simulink model "ProcessAttitude"  (R2018b)
settings: configuration reference "RPi_ControlRate" (kept outside this file)
values from neighbouring files (symbols this model uses):
  rangeTable = [2500 5000]    [loadSensorData.m]
settings Model: Creator=barthal  LastModifiedBy=barthal
settings ConfigSetRef: SourceLocation=Base Workspace

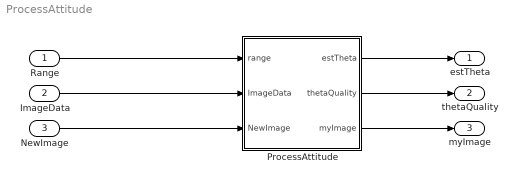
== system ProcessAttitude ==
  Range : Inport
  ImageData : Inport  Port=2  OutDataTypeStr=uint8
  NewImage : Inport  Port=3  OutDataTypeStr=uint8
  ProcessAttitude : Subsystem
  estTheta : Outport
  thetaQuality : Outport  Port=2
  myImage : Outport  Port=3  OutDataTypeStr=uint8
  wires:
  ImageData/1 -> ProcessAttitude/2(ImageData)
  Range/1 -> ProcessAttitude/1(range)
  ProcessAttitude/1(estTheta) -> estTheta/1
  ProcessAttitude/2(thetaQuality) -> thetaQuality/1
  ProcessAttitude/3(myImage) -> myImage/1
  NewImage/1 -> ProcessAttitude/3(NewImage)

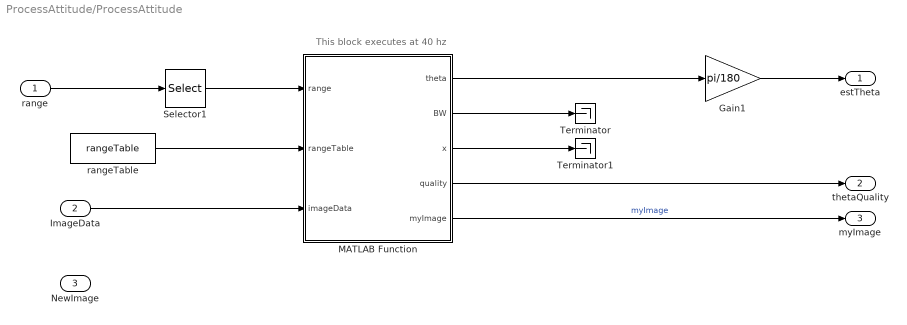
== system ProcessAttitude/ProcessAttitude ==
  note: This block executes at 40 hz
  range : Inport  PortDimensions=4
  ImageData : Inport  Port=2  OutDataTypeStr=uint8  PortDimensions=[307200]
  NewImage : Inport  Port=3
  Gain1 : Gain  Gain=pi/180
  MATLAB Function : MATLAB Function  TreatAsAtomicUnit=on
  Selector1 : Selector  InputPortWidth=4  IndexOptions=Index vector (dialog)  Indices=1  OutputSizes=1
  Terminator : Terminator
  Terminator1 : Terminator
  rangeTable : Constant  Value=rangeTable
  estTheta : Outport
  thetaQuality : Outport  Port=2
  myImage : Outport  Port=3  OutDataTypeStr=uint8
  wires:
  MATLAB Function/3(x) -> Terminator1/1
  MATLAB Function/2(BW) -> Terminator/1
  MATLAB Function/5(myImage) -> myImage/1  "myImage"
  MATLAB Function/4(quality) -> thetaQuality/1
  MATLAB Function/1(theta) -> Gain1/1
  range/1 -> Selector1/1
  Selector1/1 -> MATLAB Function/1(range)
  Gain1/1 -> estTheta/1
  rangeTable/1 -> MATLAB Function/2(rangeTable)
  ImageData/1 -> MATLAB Function/3(imageData)

== matlab function ProcessAttitude/MATLAB Function ==
  data: range input; theta output; BW output; x output; quality output; rangeTable input; imageData input; myImage output uint8
function [theta,BW,x,quality,myImage] = callimageProcess(range,rangeTable,imageData)

% persistent camObj
% 
% if isempty(camObj)
%     adaptorname = 'winvideo';
%     camObj = imaq.VideoDevice(adaptorname);
% end

% Use this if importing a 3-channel color image
% b=imageData(:,1);
% g=imageData(:,2);
% r=imageData(:,3);
% 
% b2=reshape(b,640,480);
% g2=reshape(g,640,480);
% r2=reshape(r,640,480);
% 
% myImage = uint8(zeros(480,640,3));
% 
% myImage(:,:,1) = r2';
% myImage(:,:,2) = g2';
% myImage(:,:,3) = b2';

% Use this if importing a 1 channel grayscale image
inputImage=reshape(imageData,640,480);
% myImage = uint8(zeros(480,640));
myImage = inputImage';

% theta = 0;
% BW = 0;
% x = 0;
% quality = 0;
[theta,BW,x,quality] = imageProcess(myImage,range,rangeTable);
